simulink model "exp3_2_formation_circle"  (R2020b)
settings: Solver=VariableStepAuto  StartTime=0  StopTime=50  RelTol=1e-3
values from neighbouring files (symbols this model uses):
  formation = [0,0,5,20,2]    [run_exp3_2.m]
  g = 9.8    [run_exp1.m]    (also in run_exp2.m; run_exp3_1.m; run_exp3_2.m)
  Ixx = 0.114    [run_exp1.m]    (also in run_exp2.m; run_exp3_1.m; run_exp3_2.m)
  Iyy = 0.114    [run_exp1.m]    (also in run_exp2.m; run_exp3_1.m; run_exp3_2.m)
  Izz = 0.158    [run_exp1.m]    (also in run_exp2.m; run_exp3_1.m; run_exp3_2.m)
  k_F = 6.11*10^(-8)*3600/(4*pi^2)    (= 5.57165188849e-06)    [run_exp1.m]    (also in run_exp2.m; run_exp3_1.m; run_exp3_2.m)
  k_M = 1.5*10^(-9)*3600/(4*pi^2)    (= 1.36783597917e-07)    [run_exp1.m]    (also in run_exp2.m; run_exp3_1.m; run_exp3_2.m)
  k_m = 20    [run_exp1.m]    (also in run_exp2.m; run_exp3_1.m; run_exp3_2.m)
  kd_phi = 4000    [run_exp1.m]    (also in run_exp2.m; run_exp3_1.m; run_exp3_2.m)
  kd_psi = 4000    [run_exp1.m]    (also in run_exp2.m; run_exp3_1.m; run_exp3_2.m)
  kd_theta = 4000    [run_exp1.m]    (also in run_exp2.m; run_exp3_1.m; run_exp3_2.m)
  kd_x = 1.0    (= 1)    [run_exp1.m]    (also in run_exp2.m; run_exp3_1.m; run_exp3_2.m)
  kd_y = 1.0    (= 1)    [run_exp1.m]    (also in run_exp2.m; run_exp3_1.m; run_exp3_2.m)
  kd_z = 2.0    (= 2)    [run_exp1.m]    (also in run_exp2.m; run_exp3_1.m; run_exp3_2.m)
  kp_phi = 2000    [run_exp1.m]    (also in run_exp2.m; run_exp3_1.m; run_exp3_2.m)
  kp_psi = 800    [run_exp1.m]    (also in run_exp2.m; run_exp3_1.m; run_exp3_2.m)
  kp_theta = 2000    [run_exp1.m]    (also in run_exp2.m; run_exp3_1.m; run_exp3_2.m)
  kp_x = 0.5    [run_exp1.m]    (also in run_exp2.m; run_exp3_1.m; run_exp3_2.m = 1)
  kp_y = 0.5    [run_exp1.m]    (also in run_exp2.m; run_exp3_1.m; run_exp3_2.m = 1)
  kp_z = 1.2    [run_exp1.m]    (also in run_exp2.m; run_exp3_1.m; run_exp3_2.m)
  L = 0.2    [run_exp1.m]    (also in run_exp2.m; run_exp3_1.m; run_exp3_2.m)
  m = 0.5    [run_exp1.m]    (also in run_exp2.m; run_exp3_1.m; run_exp3_2.m)
  y1_init = 0    [run_exp3_1.m]    (also in run_exp3_2.m)
  y2_init = R    (= 0.5)    [run_exp3_1.m]    (also in run_exp3_2.m = 5)
  y3_init = -R    (= -0.5)    [run_exp3_1.m]    (also in run_exp3_2.m = -5)
libraries: pid_lib x9, shared6dof x3
(part 2 of 2)

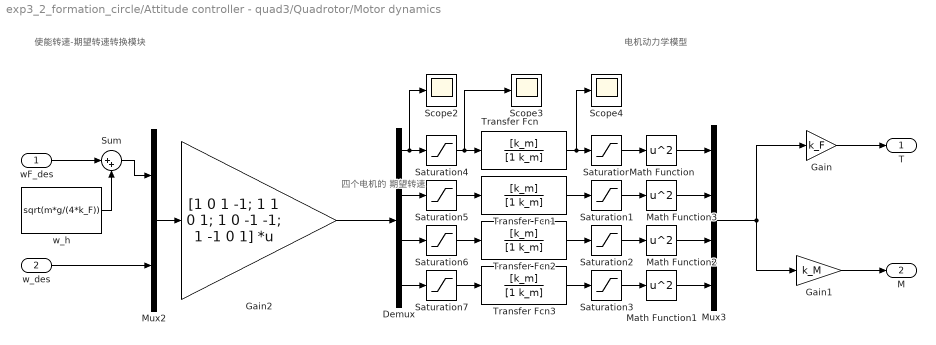
== system exp3_2_formation_circle/Attitude controller - quad3/Quadrotor/Motor dynamics ==
  note: 四个电机的
      | 期望转速
  note: 电机动力学模型
  note: 使能转速-期望转速转换模块
  wF_des : Inport
  w_des : Inport  Port=2
  Demux : Demux
  Gain : Gain  Gain=k_F
  Gain1 : Gain  Gain=k_M
  Gain2 : Gain  Gain=[1 0 1 -1; 1 1 0 1; 1 0 -1 -1; 1 -1 0 1]  Multiplication=Matrix(K*u) (u vector)
  Math Function{,1..3} (4 alike) : Math  Operator=square  SaturateOnIntegerOverflow=on
  Mux2 : Mux  Inputs=2
  Mux3 : Mux
  Saturation{,1..7} (8 alike) : Saturate  UpperLimit=7800*2*pi/60  LowerLimit=1200*2*pi/60
  Scope2 : Scope
  Scope3 : Scope
  Scope4 : Scope
  Sum : Sum  Inputs=|++
  Transfer Fcn{,1..3} (4 alike) : TransferFcn  Numerator=[k_m]  Denominator=[1 k_m]
  w_h : Constant  Value=sqrt(m*g/(4*k_F))
  T : Outport
  M : Outport  Port=2
  wires:
  Mux2/1 -> Gain2/1
  Sum/1 -> Mux2/1
  w_h/1 -> Sum/2
  Gain/1 -> T/1
  Mux3/1 -> Gain1/1, Gain/1
  Gain2/1 -> Demux/1
  Gain1/1 -> M/1
  wF_des/1 -> Sum/1
  Math Function/1 -> Mux3/1
  Math Function3/1 -> Mux3/2
  Math Function2/1 -> Mux3/3
  Math Function1/1 -> Mux3/4
  Transfer Fcn3/1 -> Saturation3/1
  Transfer Fcn/1 -> Scope4/1, Saturation/1
  Transfer Fcn1/1 -> Saturation1/1
  Transfer Fcn2/1 -> Saturation2/1
  Saturation/1 -> Math Function/1
  Saturation3/1 -> Math Function1/1
  Saturation2/1 -> Math Function2/1
  Saturation1/1 -> Math Function3/1
  w_des/1 -> Mux2/2
  Saturation6/1 -> Transfer Fcn2/1
  Saturation7/1 -> Transfer Fcn3/1
  Saturation4/1 -> Scope3/1, Transfer Fcn/1
  Saturation5/1 -> Transfer Fcn1/1
  Demux/1 -> Scope2/1, Saturation4/1
  Demux/2 -> Saturation5/1
  Demux/3 -> Saturation6/1
  Demux/4 -> Saturation7/1

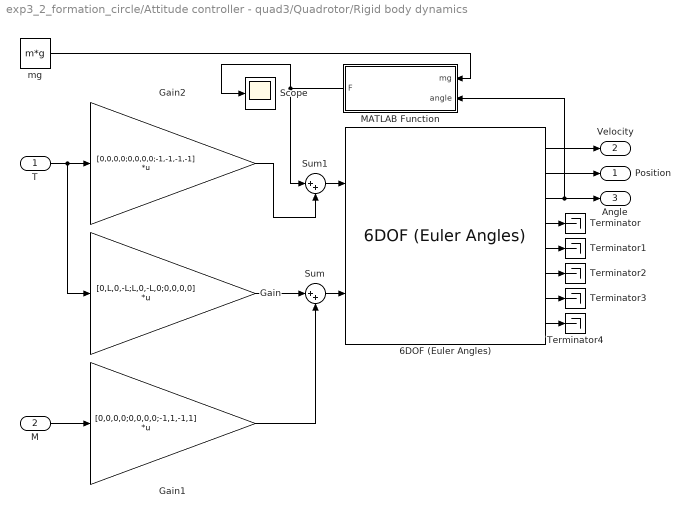
== system exp3_2_formation_circle/Attitude controller - quad3/Quadrotor/Rigid body dynamics ==
  T : Inport
  M : Inport  Port=2
  6DOF (Euler Angles) : shared6dof/6DOF (Euler Angles)  units=Metric (MKS)  mtype=Fixed  rep=Euler Angles  xme_0=[0 y3_init 0]  Vm_0=[0 0 0]  eul_0=[0 0 0]  pm_0=[0 0 0]  mass_0=m  mass_e=0.5  mass_f=2.0  inertia=[Ixx,0,0; 0,Iyy,0; 0,0,Izz]  inertia_e=eye(3)  inertia_f=2*eye(3)  k_quat=1.0  vre_flag=on  abi_flag=off  aMode=0  xme_statename=''  Vm_statename=''  eul_statename=''  quat_statename=''  pm_statename=''  mass_statename=''
      settings: SourceProductBaseCode=AE,PW,MT,UV,VE,VP
  Gain : Gain  Gain=[0,L,0,-L;L,0,-L,0;0,0,0,0]  Multiplication=Matrix(K*u) (u vector)
  Gain1 : Gain  Gain=[0,0,0,0;0,0,0,0;-1,1,-1,1]  Multiplication=Matrix(K*u) (u vector)
  Gain2 : Gain  Gain=[0,0,0,0;0,0,0,0;-1,-1,-1,-1]  Multiplication=Matrix(K*u) (u vector)
  MATLAB Function : MATLAB Function  TreatAsAtomicUnit=on
  Scope : Scope
  Sum : Sum  Inputs=|++
  Sum1 : Sum  Inputs=|++
  Terminator{,1..4} (5 alike) : Terminator
  mg : Constant  Value=m*g
  Position : Outport
  Velocity : Outport  Port=2
  Angle : Outport  Port=3
  wires:
  6DOF (Euler Angles)/1 -> Velocity/1
  T/1 -> Gain/1, Gain2/1
  6DOF (Euler Angles)/3 -> MATLAB Function/2(angle), Angle/1
  6DOF (Euler Angles)/2 -> Position/1
  Gain1/1 -> Sum/2
  Gain/1 -> Sum/1
  Sum/1 -> 6DOF (Euler Angles)/2
  M/1 -> Gain1/1
  Sum1/1 -> 6DOF (Euler Angles)/1
  Gain2/1 -> Sum1/2
  6DOF (Euler Angles)/4 -> Terminator/1
  6DOF (Euler Angles)/5 -> Terminator1/1
  6DOF (Euler Angles)/6 -> Terminator2/1
  6DOF (Euler Angles)/7 -> Terminator3/1
  6DOF (Euler Angles)/8 -> Terminator4/1
  mg/1 -> MATLAB Function/1(mg)
  MATLAB Function/1(F) -> Sum1/1, Scope/1

== matlab function exp3_2_formation_circle/Attitude controller - quad1/Quadrotor/Rigid body dynamics/MATLAB Function ==
  data: mg input; angle input; F output
function F = mg_w2b(mg, angle)
phi = angle(1);
theta = angle(2);
F = [-sin(theta);cos(theta)*sin(phi);cos(phi)*cos(theta)] * mg;
end

== matlab function exp3_2_formation_circle/Attitude controller - quad2/Quadrotor/Rigid body dynamics/MATLAB Function ==
  data: mg input; angle input; F output
function F = mg_w2b(mg, angle)
phi = angle(1);
theta = angle(2);
F = [-sin(theta);cos(theta)*sin(phi);cos(phi)*cos(theta)] * mg;
end

== matlab function exp3_2_formation_circle/Attitude controller - quad3/Quadrotor/Rigid body dynamics/MATLAB Function ==
  data: mg input; angle input; F output
function F = mg_w2b(mg, angle)
phi = angle(1);
theta = angle(2);
F = [-sin(theta);cos(theta)*sin(phi);cos(phi)*cos(theta)] * mg;
end

== matlab function exp3_2_formation_circle/formation tracker/MATLAB Function ==
  data: t input; p_des output; formation input; v_des output
function [p_des,v_des] = get_des_formation(t, formation)
% formation = [圆心x，圆心y，高度z，半径R，速度标量v] (5*1维)
agent_num = 3;
x0 = formation(1);
y0 = formation(2);
h = formation(3);
R = formation(4);
v = formation(5);
omega = v / R;

p_des = zeros(agent_num*3,1);
v_des = zeros(agent_num*3,1);

for i = 1:agent_num
    theta = omega*t + 2*pi/agent_num*(i-1);
    p_des((i-1)*3+1:i*3) = [x0 + R*cos(theta);
                            y0 + R*sin(theta);
                            h];
	v_des((i-1)*3+1:i*3) =  [-v*sin(theta);
                             v*cos(theta);
                             0];
end

end
